simulink model "Mass_spring_system"  (R2024a)
settings: Solver=VariableStepAuto  StartTime=0.0  StopTime=100  MaxStep=0.01  RelTol=1e-3
settings Model: Creator=91839
settings SolverCC: AlgebraicLoopSolver=TrustRegion
settings DataIOCC: ExternalInput=data  LoadExternalInput=on  SaveFormat=Array  DSMLogging=off  ReturnWorkspaceOutputs=off
settings DebuggingCC: UnconnectedInputMsg=warning  UnconnectedOutputMsg=warning  UnconnectedLineMsg=warning
settings ModelReferenceCC: EnableRefExpFcnMdlSchedulingChecks=on
settings SFSimCC: CustomCodeUndefinedFunction=UseInterfaceOnly
settings RTWCC: GPUComputeCapability=3.5

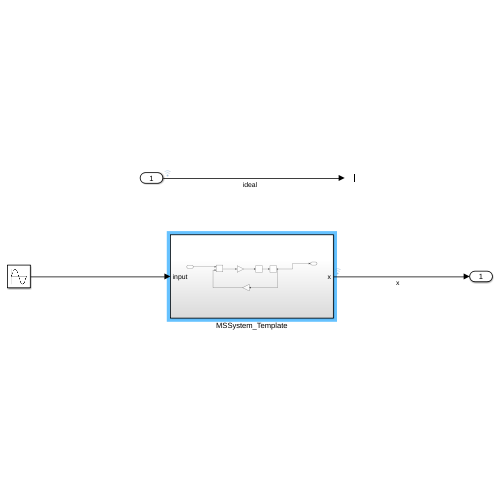
[thumbnail: Simulink's stored preview of the top-level diagram]
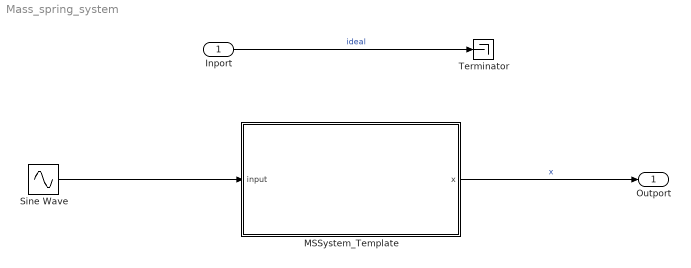
== system Mass_spring_system ==
  Inport : Inport
  MSSystem_Template : Subsystem
  Sine Wave : Sin  SampleTime=0
  Terminator : Terminator
  Outport : Outport
  wires:
  Inport/1 -> Terminator/1  "ideal"
  Sine Wave/1 -> MSSystem_Template/1(input)
  MSSystem_Template/1(x) -> Outport/1  "x"

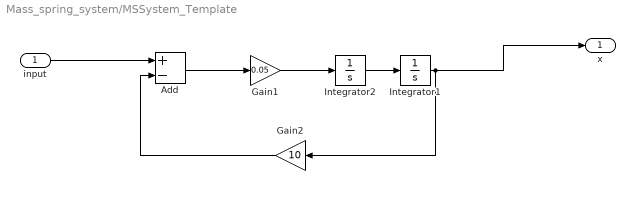
== system Mass_spring_system/MSSystem_Template ==
  input : Inport
  Add : Sum  Inputs=+-
  Gain1 : Gain  Gain=0.05
  Gain2 : Gain  Gain=10
  Integrator1 : Integrator
  Integrator2 : Integrator
  x : Outport
  wires:
  Add/1 -> Gain1/1
  Gain1/1 -> Integrator2/1
  input/1 -> Add/1
  Integrator2/1 -> Integrator1/1
  Integrator1/1 -> Gain2/1, x/1
  Gain2/1 -> Add/2
